simulink model "connections"  (R2020a)
settings: Solver=FixedStepAuto  StartTime=0.0  StopTime=5000  FixedStep=0.1  RelTol=1e-3
values from neighbouring files (symbols this model uses):
  east_drift_limit = 2    [wave_parameters.mat]
  k_down = 1.3    [wave_parameters.mat]
  k_east = 2    [wave_parameters.mat]
  k_north = 2    [wave_parameters.mat]
  k_pitch = 3    [wave_parameters.mat]
  k_roll = 3    [wave_parameters.mat]
  k_yaw = 3    [wave_parameters.mat]
  north_drift_limit = 2    [wave_parameters.mat]
  numberOfBuses = 2    [init.m]
  numberOfGenerators = 4    [init.m]
  peak_frequency = 0.8    [wave_parameters.mat]
  wave_height = 1    [wave_parameters.mat]
  yaw_drift_limit = 0.174532925199    [wave_parameters.mat]
undefined symbols (not defined in the file or in its folder): east, magnitude, north, surge, sway, yaw
libraries: simulink x28, simulink_extras x18
(part 1 of 4)
settings Model: Creator=thomas.evang  LastModifiedBy=thomas.evang
settings RTWCC: Description=Generic Real-Time Target

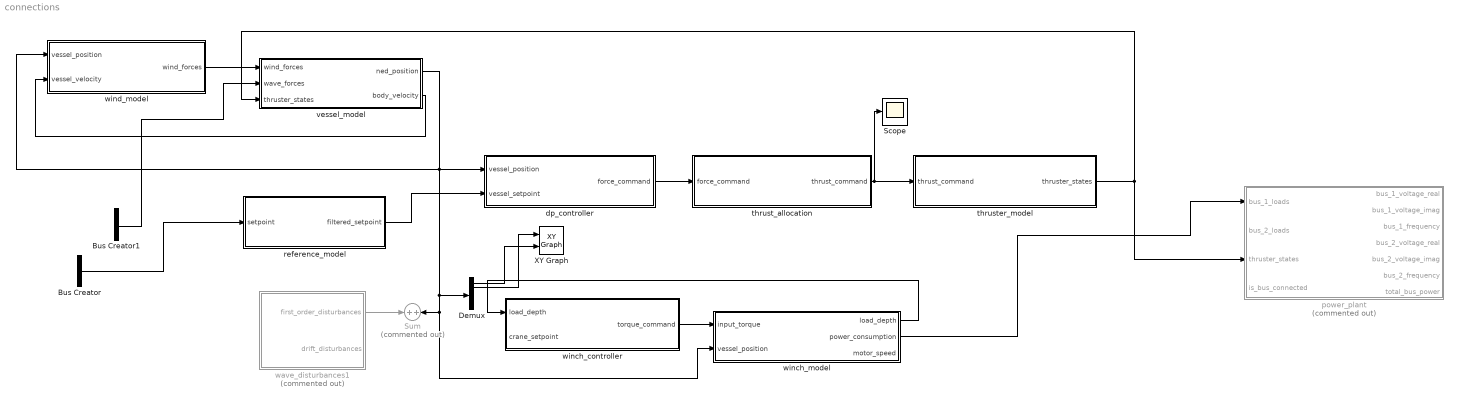
== system connections ==
  Bus Creator : BusCreator  Inputs=3  OutDataTypeStr=Bus: position_3dof
  Bus Creator1 : BusCreator  Inputs=6  OutDataTypeStr=Bus: force_6dof
  Demux : Demux  Outputs=6
  Scope : Scope
  Sum : Sum  Commented=on  Inputs=+|+
  XY Graph : simulink/Sinks/XY Graph  xmin=-20  xmax=20  ymin=-20  ymax=20  st=-1
  dp_controller : Subsystem
  power_plant : Subsystem  Commented=on
  reference_model : Subsystem
  thrust_allocation : Subsystem
  thruster_model : Subsystem
  vessel_model : Subsystem
  wave_disturbances1 : Subsystem  Commented=on  mask{Hs=wave_height, w0=peak_frequency, k_north=k_north, k_east=k_east, k_down=k_down, k_roll=k_roll, k_pitch=k_pitch, k_yaw=k_yaw}
      mask prompts: Hs "Significant Wave Height"; w0 "Peak Frequency"; k_north "North Coefficient"; k_east "East Coefficient"; k_down "Down Coefficient"; k_roll "Roll Coefficient"; k_pitch "Pitch Coefficient"; k_yaw "Yaw Coefficient"
  winch_controller : Subsystem
  winch_model : Subsystem
  wind_model : Subsystem
  wires:
  thrust_allocation/1(thrust_command) -> Scope/1, thruster_model/1(thrust_command)
  dp_controller/1(force_command) -> thrust_allocation/1(force_command)
  reference_model/1(filtered_setpoint) -> dp_controller/2(vessel_setpoint)
  thruster_model/1(thruster_states) -> vessel_model/3(thruster_states), power_plant/3(thruster_states)
  wind_model/1(wind_forces) -> vessel_model/1(wind_forces)
  vessel_model/2(body_velocity) -> wind_model/2(vessel_velocity)
  winch_controller/1(torque_command) -> winch_model/1(input_torque)
  winch_model/1(load_depth) -> winch_controller/1(load_depth)
  winch_model/2(power_consumption) -> power_plant/1(bus_1_loads)
  vessel_model/1(ned_position) -> Demux/1, winch_model/2(vessel_position), Sum/2, dp_controller/1(vessel_position), wind_model/1(vessel_position)
  wave_disturbances1/1(first_order_disturbances) -> Sum/1
  Bus Creator/1 -> reference_model/1(setpoint)
  Bus Creator1/1 -> vessel_model/2(wave_forces)
  ? -> Bus Creator/1
  Demux/2 -> XY Graph/1
  Demux/1 -> XY Graph/2

== system connections/dp_controller ==
  vessel_position : Inport  OutDataTypeStr=Bus: position_6dof
  vessel_setpoint : Inport  Port=2  OutDataTypeStr=Bus: position_3dof
  6DOFRotationMatrix : Subsystem
  Add : Sum  Inputs=-+
  Bus Creator : BusCreator  Inputs=surge,sway,yaw  OutDataTypeStr=Bus: force_3dof
  Bus to Vector : BusToVector
  Bus to Vector1 : BusToVector
  Constant1 : Constant  Value=0
  Demux : Demux  Outputs=3
  Demux1 : Demux  Outputs=3
  Demux2 : Demux  Outputs=3
  Matrix Multiply : Product  Inputs=/*  Multiplication=Matrix(*)
  PID Controller : simulink/Continuous/PID Controller  Controller=PID  Form=Parallel  TimeDomain=Discrete-time  UseExternalTs=off  SampleTime=1e-1  IntegratorMethod=Forward Euler  FilterMethod=Forward Euler  ControllerParametersSource=internal  P=10000  I=0  D=100000  UseFilter=off  N=0  TunerSelectOption=Transfer Function Based (PID Tuner App)  InitialConditionSource=internal  InitialConditionForIntegrator=0  InitialConditionForFilter=0  DifferentiatorICPrevScaledInput=0  ExternalReset=none  TrackingMode=off  Kt=1  LimitOutput=off  UpperSaturationLimit=inf  LowerSaturationLimit=-inf  LinearizeAsGain=on  AntiWindupMode=none  Kb=1  POutMin=[]  POutMax=[]  IOutMin=[]  IOutMax=[]  DOutMin=[]  DOutMax=[]  NOutMin=[]  NOutMax=[]  SumOutMin=[]  SumOutMax=[]  SaturationOutMin=[]  SaturationOutMax=[]  PParamMin=[]  PParamMax=[]  IParamMin=[]  IParamMax=[]  DParamMin=[]  DParamMax=[]  NParamMin=[]  NParamMax=[]  KbParamMin=[]  KbParamMax=[]  KtParamMin=[]  KtParamMax=[]  KbOutMin=[]  KbOutMax=[]  KtOutMin=[]  KtOutMax=[]  IntegratorOutMin=[]  IntegratorOutMax=[]  FilterOutMin=[]  FilterOutMax=[]  SumI1OutMin=[]  SumI1OutMax=[]  SumI2OutMin=[]  SumI2OutMax=[]  SumI3OutMin=[]  SumI3OutMax=[]  SumI4OutMin=[]  SumI4OutMax=[]  SumDOutMin=[]  SumDOutMax=[]  DifferentiatorOutMin=[]  DifferentiatorOutMax=[]  FilterDiffOutCoefMin=[]  FilterDiffOutCoefMax=[]  ReciprocalOutMin=[]  ReciprocalOutMax=[]  SumDenOutMin=[]  SumDenOutMax=[]  SumNumOutMin=[]  SumNumOutMax=[]  DivideOutMin=[]  DivideOutMax=[]  UdiffTsProdOutMin=[]  UdiffTsProdOutMax=[]  NTsProdOutMin=[]  NTsProdOutMax=[]  UintegralTsProdOutMin=[]  UintegralTsProdOutMax=[]  UngainTsProdOutMin=[]  UngainTsProdOutMax=[]  IntegratorContinuousStateAttributes=''  IntegratorStateMustResolveToSignalObject=off  IntegratorRTWStateStorageClass=Auto  FilterContinuousStateAttributes=''  FilterStateMustResolveToSignalObject=off  FilterRTWStateStorageClass=Auto  ParallelPVariant=InternalParameters  IdealPVariant=Disabled  IVariant=InternalParameters  DVariant=InternalParameters  IntegratorVariant=Discrete  SatVariant=Disabled  AWVariant=Passthrough  PCopyVariant=Disabled  TRVariant=Disabled  FdbkBlocksVariant=Forward  IdealPFdbkVariant=Disabled  SatFdbkVariant=Disabled  DerivativeFilterVariant=Differentiator  NVariant=Passthrough  NCopyVariant=Disabled_SignalSpec  FilterICVariant=InternalICsDifferentiator  IntegratorICVariant=InternalICs  ExternalResetVariant=Disabled  TRSumVariant=Passthrough  SumFdbkVariant=Disabled  SumVariant=Sum_PID  TsampFilterVariant=InternalTs  TsampNgainVariant=Passthrough  TsampIntegralVariant=Passthrough
  PID Controller1 : simulink/Continuous/PID Controller  Controller=PID  Form=Parallel  TimeDomain=Discrete-time  UseExternalTs=off  SampleTime=1e-1  IntegratorMethod=Forward Euler  FilterMethod=Forward Euler  ControllerParametersSource=internal  P=10000  I=0  D=100000  UseFilter=off  N=0  TunerSelectOption=Transfer Function Based (PID Tuner App)  InitialConditionSource=internal  InitialConditionForIntegrator=0  InitialConditionForFilter=0  DifferentiatorICPrevScaledInput=0  ExternalReset=none  TrackingMode=off  Kt=1  LimitOutput=off  UpperSaturationLimit=inf  LowerSaturationLimit=-inf  LinearizeAsGain=on  AntiWindupMode=none  Kb=1  POutMin=[]  POutMax=[]  IOutMin=[]  IOutMax=[]  DOutMin=[]  DOutMax=[]  NOutMin=[]  NOutMax=[]  SumOutMin=[]  SumOutMax=[]  SaturationOutMin=[]  SaturationOutMax=[]  PParamMin=[]  PParamMax=[]  IParamMin=[]  IParamMax=[]  DParamMin=[]  DParamMax=[]  NParamMin=[]  NParamMax=[]  KbParamMin=[]  KbParamMax=[]  KtParamMin=[]  KtParamMax=[]  KbOutMin=[]  KbOutMax=[]  KtOutMin=[]  KtOutMax=[]  IntegratorOutMin=[]  IntegratorOutMax=[]  FilterOutMin=[]  FilterOutMax=[]  SumI1OutMin=[]  SumI1OutMax=[]  SumI2OutMin=[]  SumI2OutMax=[]  SumI3OutMin=[]  SumI3OutMax=[]  SumI4OutMin=[]  SumI4OutMax=[]  SumDOutMin=[]  SumDOutMax=[]  DifferentiatorOutMin=[]  DifferentiatorOutMax=[]  FilterDiffOutCoefMin=[]  FilterDiffOutCoefMax=[]  ReciprocalOutMin=[]  ReciprocalOutMax=[]  SumDenOutMin=[]  SumDenOutMax=[]  SumNumOutMin=[]  SumNumOutMax=[]  DivideOutMin=[]  DivideOutMax=[]  UdiffTsProdOutMin=[]  UdiffTsProdOutMax=[]  NTsProdOutMin=[]  NTsProdOutMax=[]  UintegralTsProdOutMin=[]  UintegralTsProdOutMax=[]  UngainTsProdOutMin=[]  UngainTsProdOutMax=[]  IntegratorContinuousStateAttributes=''  IntegratorStateMustResolveToSignalObject=off  IntegratorRTWStateStorageClass=Auto  FilterContinuousStateAttributes=''  FilterStateMustResolveToSignalObject=off  FilterRTWStateStorageClass=Auto  ParallelPVariant=InternalParameters  IdealPVariant=Disabled  IVariant=InternalParameters  DVariant=InternalParameters  IntegratorVariant=Discrete  SatVariant=Disabled  AWVariant=Passthrough  PCopyVariant=Disabled  TRVariant=Disabled  FdbkBlocksVariant=Forward  IdealPFdbkVariant=Disabled  SatFdbkVariant=Disabled  DerivativeFilterVariant=Differentiator  NVariant=Passthrough  NCopyVariant=Disabled_SignalSpec  FilterICVariant=InternalICsDifferentiator  IntegratorICVariant=InternalICs  ExternalResetVariant=Disabled  TRSumVariant=Passthrough  SumFdbkVariant=Disabled  SumVariant=Sum_PID  TsampFilterVariant=InternalTs  TsampNgainVariant=Passthrough  TsampIntegralVariant=Passthrough
  PID Controller2 : simulink/Continuous/PID Controller  Controller=PID  Form=Parallel  TimeDomain=Discrete-time  UseExternalTs=off  SampleTime=1e-1  IntegratorMethod=Forward Euler  FilterMethod=Forward Euler  ControllerParametersSource=internal  P=10000  I=10  D=100000  UseFilter=off  N=100  TunerSelectOption=Transfer Function Based (PID Tuner App)  InitialConditionSource=internal  InitialConditionForIntegrator=0  InitialConditionForFilter=0  DifferentiatorICPrevScaledInput=0  ExternalReset=none  TrackingMode=off  Kt=1  LimitOutput=off  UpperSaturationLimit=inf  LowerSaturationLimit=-inf  LinearizeAsGain=on  AntiWindupMode=none  Kb=1  POutMin=[]  POutMax=[]  IOutMin=[]  IOutMax=[]  DOutMin=[]  DOutMax=[]  NOutMin=[]  NOutMax=[]  SumOutMin=[]  SumOutMax=[]  SaturationOutMin=[]  SaturationOutMax=[]  PParamMin=[]  PParamMax=[]  IParamMin=[]  IParamMax=[]  DParamMin=[]  DParamMax=[]  NParamMin=[]  NParamMax=[]  KbParamMin=[]  KbParamMax=[]  KtParamMin=[]  KtParamMax=[]  KbOutMin=[]  KbOutMax=[]  KtOutMin=[]  KtOutMax=[]  IntegratorOutMin=[]  IntegratorOutMax=[]  FilterOutMin=[]  FilterOutMax=[]  SumI1OutMin=[]  SumI1OutMax=[]  SumI2OutMin=[]  SumI2OutMax=[]  SumI3OutMin=[]  SumI3OutMax=[]  SumI4OutMin=[]  SumI4OutMax=[]  SumDOutMin=[]  SumDOutMax=[]  DifferentiatorOutMin=[]  DifferentiatorOutMax=[]  FilterDiffOutCoefMin=[]  FilterDiffOutCoefMax=[]  ReciprocalOutMin=[]  ReciprocalOutMax=[]  SumDenOutMin=[]  SumDenOutMax=[]  SumNumOutMin=[]  SumNumOutMax=[]  DivideOutMin=[]  DivideOutMax=[]  UdiffTsProdOutMin=[]  UdiffTsProdOutMax=[]  NTsProdOutMin=[]  NTsProdOutMax=[]  UintegralTsProdOutMin=[]  UintegralTsProdOutMax=[]  UngainTsProdOutMin=[]  UngainTsProdOutMax=[]  IntegratorContinuousStateAttributes=''  IntegratorStateMustResolveToSignalObject=off  IntegratorRTWStateStorageClass=Auto  FilterContinuousStateAttributes=''  FilterStateMustResolveToSignalObject=off  FilterRTWStateStorageClass=Auto  ParallelPVariant=InternalParameters  IdealPVariant=Disabled  IVariant=InternalParameters  DVariant=InternalParameters  IntegratorVariant=Discrete  SatVariant=Disabled  AWVariant=Passthrough  PCopyVariant=Disabled  TRVariant=Disabled  FdbkBlocksVariant=Forward  IdealPFdbkVariant=Disabled  SatFdbkVariant=Disabled  DerivativeFilterVariant=Differentiator  NVariant=Passthrough  NCopyVariant=Disabled_SignalSpec  FilterICVariant=InternalICsDifferentiator  IntegratorICVariant=InternalICs  ExternalResetVariant=Disabled  TRSumVariant=Passthrough  SumFdbkVariant=Disabled  SumVariant=Sum_PID  TsampFilterVariant=InternalTs  TsampNgainVariant=Passthrough  TsampIntegralVariant=Passthrough
  Scope : Scope
  Scope1 : Scope
  Scope2 : Scope
  Selector1 : Selector  InputPortWidth=6  IndexOptions=Index vector (dialog)  Indices=[1 2 6]  OutputSizes=1
  Selector2 : Selector  InputPortWidth=6  IndexOptions=Index vector (dialog)  Indices=[1 2 6]  OutputSizes=1
  Selector3 : Selector  InputPortWidth=6  IndexOptions=Index vector (dialog)  Indices=[4 5 6]  OutputSizes=1
  Vector Concatenate : Concatenate  NumInputs=6
  force_command : Outport  OutDataTypeStr=Bus: force_3dof  VectorParamsAs1DForOutWhenUnconnected=off
  wires:
  vessel_position/1 -> Bus to Vector/1
  Selector2/1 -> Demux1/1
  Bus to Vector/1 -> Selector3/1, Selector1/1
  PID Controller1/1 -> Vector Concatenate/2
  Matrix Multiply/1 -> Selector2/1
  Demux1/3 -> Bus Creator/3  "yaw"
  Bus to Vector1/1 -> Add/2
  Selector1/1 -> Add/1
  Demux/1 -> PID Controller/1, Scope1/1  "errorN"
  Demux/2 -> Scope2/1, PID Controller1/1  "errorE"
  Constant1/1 -> Vector Concatenate/5, Vector Concatenate/3, Vector Concatenate/4
  PID Controller2/1 -> Vector Concatenate/6
  6DOFRotationMatrix/1(6DofRotationMatrix) -> Matrix Multiply/1
  Demux1/2 -> Bus Creator/2  "sway"
  Demux/3 -> Scope/1, PID Controller2/1  "errorHeading"
  Bus Creator/1 -> force_command/1
  vessel_setpoint/1 -> Bus to Vector1/1
  Demux1/1 -> Bus Creator/1  "surge"
  Vector Concatenate/1 -> Matrix Multiply/2
  Add/1 -> Demux/1
  PID Controller/1 -> Vector Concatenate/1
  Selector3/1 -> Demux2/1
  Demux2/1 -> 6DOFRotationMatrix/1(roll)
  Demux2/2 -> 6DOFRotationMatrix/2(pitch)
  Demux2/3 -> 6DOFRotationMatrix/3(yaw)

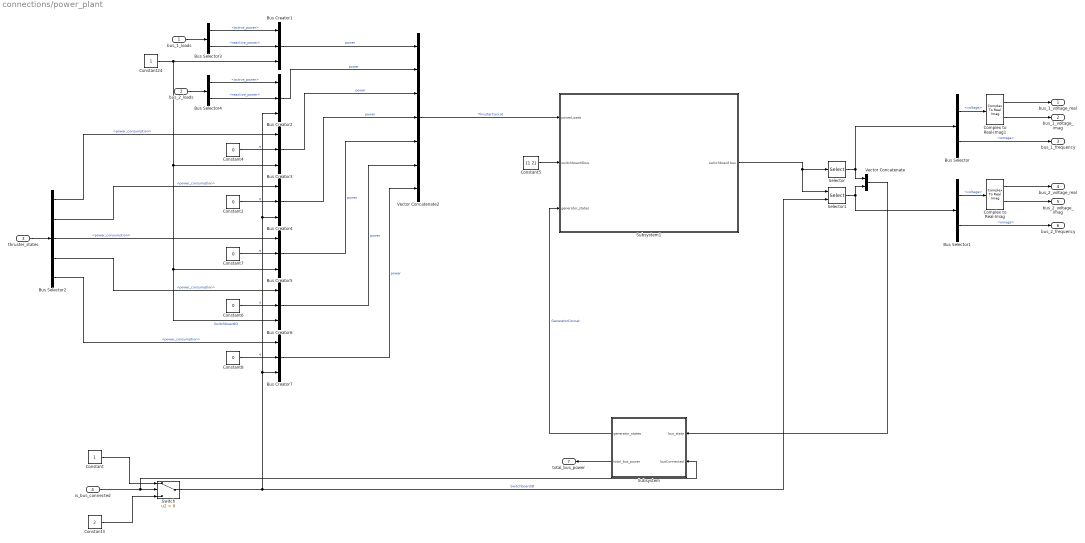
== system connections/power_plant ==
  bus_1_loads : Inport  OutDataTypeStr=Bus: bus_load
  bus_2_loads : Inport  Port=2  OutDataTypeStr=Bus: bus_load
  thruster_states : Inport  Port=3  OutDataTypeStr=Bus: thruster_states
  is_bus_connected : Inport  Port=4  OutDataTypeStr=boolean
  Bus Selector : BusSelector  OutputSignals=voltage,omega
  Bus Selector1 : BusSelector  OutputSignals=voltage,omega
  Bus Selector2 : BusSelector  OutputSignals=tunnel_thruster_1.power_consumption,tunnel_thruster_2.power_consumption,tunnel_thruster_3.power_consumption,main_propeller_port.power_consumption,main_propeller_starboard.power_consumption
  Bus Selector3 : BusSelector  OutputSignals=active_power,reactive_power
  Bus Selector4 : BusSelector  OutputSignals=active_power,reactive_power
  Bus Creator{1..7} (7 alike) : BusCreator  Inputs=3  OutDataTypeStr=Bus: powerLoadsBus  NonVirtualBus=on
      settings: InheritFromInputs=off
  Complex to Real-Imag : ComplexToRealImag
  Complex to Real-Imag1 : ComplexToRealImag
  Constant : Constant
  Constant{2,4,6..8} (5 alike) : Constant  Value=0
  Constant24 : Constant
  Constant3 : Constant  Value=2
  Constant5 : Constant  Value=[1 2]
  Selector : Selector  NumberOfDimensions=2  InputPortWidth=3  IndexOptions=Select all,Index vector (dialog)  Indices=[1 3],1  OutputSizes=1,1
  Selector1 : Selector  NumberOfDimensions=2  InputPortWidth=3  IndexOptions=Select all,Index vector (port)  Indices=[1 3],1  OutputSizes=1,1
  Subsystem : Subsystem
  Subsystem1 : Subsystem
  Switch : Switch  Criteria=u2 > Threshold
  Vector Concatenate : Concatenate  Mode=Multidimensional array  ConcatenateDimension=2
  Vector Concatenate2 : Concatenate  NumInputs=7  Mode=Multidimensional array
  bus_1_voltage_real : Outport  OutDataTypeStr=double  VectorParamsAs1DForOutWhenUnconnected=off
  bus_1_voltage_imag : Outport  Port=2  OutDataTypeStr=double  VectorParamsAs1DForOutWhenUnconnected=off
  bus_1_frequency : Outport  Port=3  OutDataTypeStr=double  VectorParamsAs1DForOutWhenUnconnected=off
  bus_2_voltage_real : Outport  Port=4  OutDataTypeStr=double  VectorParamsAs1DForOutWhenUnconnected=off
  bus_2_voltage_imag : Outport  Port=5  OutDataTypeStr=double  VectorParamsAs1DForOutWhenUnconnected=off
  bus_2_frequency : Outport  Port=6  OutDataTypeStr=double  VectorParamsAs1DForOutWhenUnconnected=off
  total_bus_power : Outport  Port=7  OutDataTypeStr=double  VectorParamsAs1DForOutWhenUnconnected=off
  wires:
  Selector1/1 -> Vector Concatenate/2, Bus Selector1/1
  Bus Selector/1 -> Complex to Real-Imag1/1  "<voltage>"
  Constant24/1 -> Bus Creator6/3, Bus Creator5/3, Bus Creator3/3, Bus Creator1/3  "SwitchboardID"
  Switch/1 -> Bus Creator2/3, Bus Creator4/3, Bus Creator7/3, Selector1/2  "SwitchboardID"
  Constant/1 -> Switch/1
  Subsystem/1(generator_states) -> Subsystem1/3(generator_states)  "GeneratorConcat"
  Bus Creator1/1 -> Vector Concatenate2/1  "power"
  Vector Concatenate2/1 -> Subsystem1/1(powerLoads)  "ThrusterConcat"
  Bus Selector1/2 -> bus_2_frequency/1  "<omega>"
  Subsystem/2(total_bus_power) -> total_bus_power/1
  bus_1_loads/1 -> Bus Selector3/1
  Constant4/1 -> Bus Creator3/2  "q"
  Constant6/1 -> Bus Creator6/2  "q"
  Bus Selector3/1 -> Bus Creator1/1  "<active_power>"
  is_bus_connected/1 -> Subsystem/2(busConnected), Switch/2
  Bus Creator7/1 -> Vector Concatenate2/7  "power"
  bus_2_loads/1 -> Bus Selector4/1
  Subsystem1/1(switchboard bus) -> Selector/1, Selector1/1
  Constant5/1 -> Subsystem1/2(switchboard2bus)
  Bus Selector3/2 -> Bus Creator1/2  "<reactive_power>"
  Bus Selector1/1 -> Complex to Real-Imag/1  "<voltage>"
  Bus Selector2/3 -> Bus Creator5/1  "<power_consumption>"
  Bus Selector2/4 -> Bus Creator6/1  "<power_consumption>"
  Bus Selector4/2 -> Bus Creator2/2  "<reactive_power>"
  Bus Selector2/2 -> Bus Creator4/1  "<power_consumption>"
  Bus Selector2/1 -> Bus Creator3/1  "<power_consumption>"
  Selector/1 -> Vector Concatenate/1, Bus Selector/1
  Vector Concatenate/1 -> Subsystem/1(bus_state)
  Bus Creator6/1 -> Vector Concatenate2/6  "power"
  Bus Creator5/1 -> Vector Concatenate2/5  "power"
  Complex to Real-Imag1/1 -> bus_1_voltage_real/1
  Bus Selector/2 -> bus_1_frequency/1  "<omega>"
  Constant8/1 -> Bus Creator7/2  "q"
  thruster_states/1 -> Bus Selector2/1
  Complex to Real-Imag/2 -> bus_2_voltage_imag/1
  Constant7/1 -> Bus Creator5/2  "q"
  Constant3/1 -> Switch/3
  Bus Creator3/1 -> Vector Concatenate2/3  "power"
  Constant2/1 -> Bus Creator4/2  "q"
  Bus Creator4/1 -> Vector Concatenate2/4  "power"
  Complex to Real-Imag1/2 -> bus_1_voltage_imag/1
  Bus Selector2/5 -> Bus Creator7/1  "<power_consumption>"
  Complex to Real-Imag/1 -> bus_2_voltage_real/1
  Bus Creator2/1 -> Vector Concatenate2/2  "power"
  Bus Selector4/1 -> Bus Creator2/1  "<active_power>"

== system connections/reference_model ==
  setpoint : Inport  OutDataTypeStr=Bus: position_3dof
  Add1 : Sum  Inputs=|+-
  Add2 : Sum  Inputs=|+-
  Bus Creator : BusCreator  Inputs=north,east,yaw  OutDataTypeStr=Bus: position_3dof
  Bus to Vector : BusToVector
  Demux : Demux  Outputs=3
  Gain1 : Gain  Gain=[10 10 20].*[10 10 20]
  Gain2 : Gain  Gain=2*[10 10 20]
  Gain3 : Gain  Gain=[10 10 20].*[10 10 20]
  Integrator : Integrator  InitialCondition=0*1*[1 1 1]  ZeroCross=off
  Integrator1 : Integrator  InitialCondition=0*1*[1 1 1]  ZeroCross=off
  Saturation : Saturate  UpperLimit=1*[1 1 pi/18/6]  LowerLimit=-1*[1 1 pi/18/6]  ZeroCross=off
  Saturation1 : Saturate  UpperLimit=1*[5 5 1]  LowerLimit=-1*[5 5 1]  ZeroCross=off
  filtered_setpoint : Outport  OutDataTypeStr=Bus: position_3dof  VectorParamsAs1DForOutWhenUnconnected=off
  wires:
  Demux/1 -> Bus Creator/1  "north"
  Integrator1/1 -> Gain3/1, Demux/1
  Gain1/1 -> Add2/1
  Saturation1/1 -> Integrator/1
  Add2/1 -> Add1/1
  Saturation/1 -> Integrator1/1
  Integrator/1 -> Gain2/1, Saturation/1
  Gain2/1 -> Add1/2
  Demux/3 -> Bus Creator/3  "yaw"
  Add1/1 -> Saturation1/1
  Gain3/1 -> Add2/2
  Bus to Vector/1 -> Gain1/1
  Demux/2 -> Bus Creator/2  "east"
  setpoint/1 -> Bus to Vector/1
  Bus Creator/1 -> filtered_setpoint/1

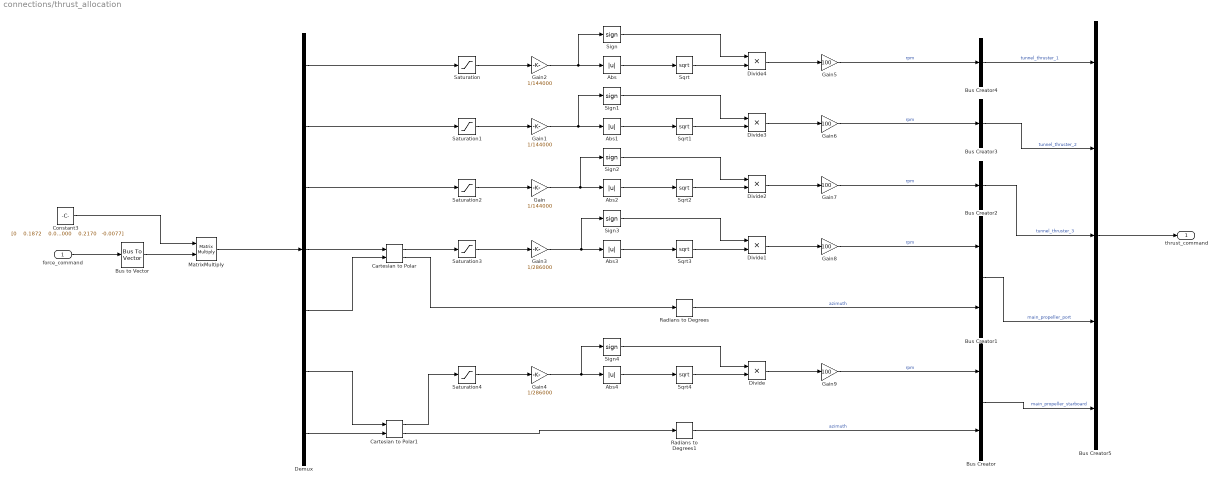
== system connections/thrust_allocation ==
  force_command : Inport  OutDataTypeStr=Bus: force_3dof
  Abs{,1..4} (5 alike) : Abs
  Bus Creator : BusCreator  Inputs=2  OutDataTypeStr=Bus: azimuth_thruster_command
      settings: InheritFromInputs=off
  Bus Creator1 : BusCreator  Inputs=2  OutDataTypeStr=Bus: azimuth_thruster_command
      settings: InheritFromInputs=off
  Bus Creator2 : BusCreator  Inputs=1  OutDataTypeStr=Bus: tunnel_thruster_command
      settings: InheritFromInputs=off
  Bus Creator3 : BusCreator  Inputs=1  OutDataTypeStr=Bus: tunnel_thruster_command
      settings: InheritFromInputs=off
  Bus Creator4 : BusCreator  Inputs=1  OutDataTypeStr=Bus: tunnel_thruster_command
      settings: InheritFromInputs=off
  Bus Creator5 : BusCreator  Inputs=5  OutDataTypeStr=Bus: thrust_command
      settings: InheritFromInputs=off
  Bus to Vector : BusToVector
  Cartesian to Polar : simulink_extras/Transformations/Cartesian to Polar
  Cartesian to Polar1 : simulink_extras/Transformations/Cartesian to Polar
  Constant3 : Constant  Value=|
      | [0    0.1872    0.0058;
      |     0.0000    0.1886    0.0051;
      |     0.0000    0.1901    0.0045;
      |     0.5000   -0.0018    0.0008;
      |     0.0000    0.2170   -0.0077;
      |     0.5000    0.0018   -0.0008;
      |     0.0000    0.2170   -0.0077]
  Demux : Demux  Outputs=7
  Divide{,1..4} (5 alike) : Product
  Gain : Gain  Gain=1/144000
  Gain1 : Gain  Gain=1/144000
  Gain2 : Gain  Gain=1/144000
  Gain3 : Gain  Gain=1/286000
  Gain4 : Gain  Gain=1/286000
  Gain{5..9} (5 alike) : Gain  Gain=100
  MatrixMultiply : Product  Multiplication=Matrix(*)
  Radians to Degrees : simulink_extras/Transformations/Radians to Degrees
  Radians to Degrees1 : simulink_extras/Transformations/Radians to Degrees
  Saturation : Saturate  UpperLimit=144000  LowerLimit=-144000
  Saturation1 : Saturate  UpperLimit=144000  LowerLimit=-144000
  Saturation2 : Saturate  UpperLimit=144000  LowerLimit=-144000
  Saturation3 : Saturate  UpperLimit=286000  LowerLimit=0
  Saturation4 : Saturate  UpperLimit=286000  LowerLimit=0
  Sign{,1..4} (5 alike) : Signum
  Sqrt{,1..4} (5 alike) : Sqrt  SaturateOnIntegerOverflow=on
  thrust_command : Outport  OutDataTypeStr=Bus: thrust_command  VectorParamsAs1DForOutWhenUnconnected=off
  wires:
  Saturation2/1 -> Gain/1
  Constant3/1 -> MatrixMultiply/1
  Abs1/1 -> Sqrt1/1
  MatrixMultiply/1 -> Demux/1
  Gain1/1 -> Sign1/1, Abs1/1
  Saturation3/1 -> Gain3/1
  Gain2/1 -> Sign/1, Abs/1
  Sign2/1 -> Divide2/1
  Sign/1 -> Divide4/1
  Bus Creator5/1 -> thrust_command/1
  Demux/2 -> Saturation1/1
  Bus to Vector/1 -> MatrixMultiply/2
  Saturation1/1 -> Gain1/1
  Bus Creator3/1 -> Bus Creator5/2  "tunnel_thruster_2"
  Bus Creator2/1 -> Bus Creator5/3  "tunnel_thruster_3"
  Bus Creator4/1 -> Bus Creator5/1  "tunnel_thruster_1"
  Abs4/1 -> Sqrt4/1
  Sqrt/1 -> Divide4/2
  Demux/1 -> Saturation/1
  Bus Creator/1 -> Bus Creator5/5  "main_propeller_starboard"
  Gain/1 -> Sign2/1, Abs2/1
  Demux/4 -> Cartesian to Polar/1
  Sqrt1/1 -> Divide3/2
  Sign4/1 -> Divide/1
  Gain8/1 -> Bus Creator1/1  "rpm"
  Gain5/1 -> Bus Creator4/1  "rpm"
  Divide1/1 -> Gain8/1
  Gain6/1 -> Bus Creator3/1  "rpm"
  force_command/1 -> Bus to Vector/1
  Cartesian to Polar/1 -> Saturation3/1
  Sqrt2/1 -> Divide2/2
  Abs3/1 -> Sqrt3/1
  Cartesian to Polar1/1 -> Saturation4/1
  Divide2/1 -> Gain7/1
  Gain3/1 -> Sign3/1, Abs3/1
  Gain9/1 -> Bus Creator/1  "rpm"
  Sign1/1 -> Divide3/1
  Radians to Degrees1/1 -> Bus Creator/2  "azimuth"
  Demux/5 -> Cartesian to Polar/2
  Demux/6 -> Cartesian to Polar1/1
  Bus Creator1/1 -> Bus Creator5/4  "main_propeller_port"
  Demux/3 -> Saturation2/1
  Divide3/1 -> Gain6/1
  Sqrt3/1 -> Divide1/2
  Divide/1 -> Gain9/1
  Divide4/1 -> Gain5/1
  Saturation/1 -> Gain2/1
  Radians to Degrees/1 -> Bus Creator1/2  "azimuth"
  Demux/7 -> Cartesian to Polar1/2
  Abs2/1 -> Sqrt2/1
  Gain4/1 -> Sign4/1, Abs4/1
  Sqrt4/1 -> Divide/2
  Abs/1 -> Sqrt/1
  Saturation4/1 -> Gain4/1
  Gain7/1 -> Bus Creator2/1  "rpm"
  Sign3/1 -> Divide1/1
  Cartesian to Polar1/2 -> Radians to Degrees1/1
  Cartesian to Polar/2 -> Radians to Degrees/1

== system connections/thruster_model ==
  note: MPPS
  note: TT1
  note: TT1
  note: TT3
  note: TT2
  note: MPSB
  thrust_command : Inport  OutDataTypeStr=Bus: thrust_command
  Bus Creator : BusCreator  Inputs=3
  Bus Creator1 : BusCreator  Inputs=3
  Bus Creator2 : BusCreator  Inputs=2
  Bus Creator3 : BusCreator  Inputs=2
  Bus Creator4 : BusCreator  Inputs=2
  Bus Creator5 : BusCreator  Inputs=5  OutDataTypeStr=Bus: thruster_states
  Bus to Vector : BusToVector
  Constant : Constant  Value=90
  Demux : Demux  Outputs=7
  Terminator{,1..7} (8 alike) : Terminator
  main_propeller_port : Subsystem
  main_propeller_starboard : Subsystem
  tunnel_thruster_1 : Subsystem
  tunnel_thruster_2 : Subsystem
  tunnel_thruster_3 : Subsystem
  thruster_states : Outport  OutDataTypeStr=Bus: thruster_states  VectorParamsAs1DForOutWhenUnconnected=off
  wires:
  tunnel_thruster_1/2(thrust) -> Bus Creator4/2  "thrust"
  main_propeller_starboard/1(p) -> Bus Creator1/1  "power_consumption"
  Bus Creator3/1 -> Bus Creator5/2  "tunnel_thruster_2"
  Demux/7 -> main_propeller_starboard/2(desiredAzimuth)
  Bus Creator2/1 -> Bus Creator5/3  "tunnel_thruster_3"
  main_propeller_starboard/3(azimuth) -> Bus Creator1/3  "azimuth"
  tunnel_thruster_1/3(azimuth) -> Terminator6/1
  main_propeller_port/2(thrust) -> Bus Creator/2  "thrust"
  tunnel_thruster_2/2(thrust) -> Bus Creator3/2  "thrust"
  tunnel_thruster_1/1(p) -> Bus Creator4/1  "power_consumption"
  Demux/3 -> tunnel_thruster_3/1(desiredSetPoint)
  Demux/6 -> main_propeller_starboard/1(desiredSetPoint)
  Bus Creator4/1 -> Bus Creator5/1  "tunnel_thruster_1"
  tunnel_thruster_1/4(sensorFeedback) -> Terminator7/1
  tunnel_thruster_3/1(p) -> Bus Creator2/1  "power_consumption"
  tunnel_thruster_2/1(p) -> Bus Creator3/1  "power_consumption"
  main_propeller_port/1(p) -> Bus Creator/1  "power_consumption"
  tunnel_thruster_3/2(thrust) -> Bus Creator2/2  "thrust"
  Bus Creator1/1 -> Bus Creator5/5  "main_propeller_starboard"
  tunnel_thruster_3/3(azimuth) -> Terminator2/1
  Bus Creator/1 -> Bus Creator5/4  "main_propeller_port"
  Demux/2 -> tunnel_thruster_2/1(desiredSetPoint)
  main_propeller_port/3(azimuth) -> Bus Creator/3  "azimuth"
  main_propeller_port/4(sensorFeedback) -> Terminator1/1
  Bus Creator5/1 -> thruster_states/1
  main_propeller_starboard/4(sensorFeedback) -> Terminator/1
  tunnel_thruster_2/4(sensorFeedback) -> Terminator5/1
  Demux/5 -> main_propeller_port/2(desiredAzimuth)
  thrust_command/1 -> Bus to Vector/1
  tunnel_thruster_3/4(sensorFeedback) -> Terminator3/1
  main_propeller_starboard/2(thrust) -> Bus Creator1/2  "thrust"
  Demux/4 -> main_propeller_port/1(desiredSetPoint)
  Constant/1 -> tunnel_thruster_3/2(desiredAzimuth), tunnel_thruster_2/2(desiredAzimuth), tunnel_thruster_1/2(desiredAzimuth)
  Bus to Vector/1 -> Demux/1
  Demux/1 -> tunnel_thruster_1/1(desiredSetPoint)
  tunnel_thruster_2/3(azimuth) -> Terminator4/1

== system connections/vessel_model ==
  wind_forces : Inport  OutDataTypeStr=Bus: force_6dof
  wave_forces : Inport  Port=2  OutDataTypeStr=Bus: force_6dof
  thruster_states : Inport  Port=3  OutDataTypeStr=Bus: thruster_states
  Add : Sum  Inputs=+++|
  Bus Creator : BusCreator  Inputs=6  OutDataTypeStr=Bus: position_6dof
  Bus Creator2 : BusCreator  Inputs=6  OutDataTypeStr=Bus: velocity_6dof
  Bus Selector : BusSelector  OutputSignals=tunnel_thruster_1,tunnel_thruster_2,tunnel_thruster_3,main_propeller_port,main_propeller_starboard
  Bus to Vector : BusToVector
  Bus to Vector1 : BusToVector
  Demux : Demux  Outputs=6
  Demux1 : Demux  Outputs=6
  VesselDynamics : Subsystem
  thrust_to_forces : Subsystem
  ned_position : Outport  OutDataTypeStr=Bus: position_6dof  VectorParamsAs1DForOutWhenUnconnected=off
  body_velocity : Outport  Port=2  OutDataTypeStr=Bus: velocity_6dof  VectorParamsAs1DForOutWhenUnconnected=off
  wires:
  thrust_to_forces/1(ForcesAndMomentsvector) -> Add/3
  thruster_states/1 -> Bus Selector/1
  Bus Selector/5 -> thrust_to_forces/5(main_propeller_starboard)  "<main_propeller_starboard>"
  Demux1/2 -> Bus Creator2/2
  Add/1 -> VesselDynamics/1(ExternalForceAndMoments)
  Demux/1 -> Bus Creator/1
  Demux/5 -> Bus Creator/5
  Bus Selector/3 -> thrust_to_forces/3(tunnel_thruster_3)  "<tunnel_thruster_3>"
  Demux1/5 -> Bus Creator2/5
  Bus Selector/1 -> thrust_to_forces/1(tunnel_thruster_1)  "<tunnel_thruster_1>"
  Bus Creator/1 -> ned_position/1
  Demux/4 -> Bus Creator/4
  Bus Creator2/1 -> body_velocity/1
  Bus Selector/2 -> thrust_to_forces/2(tunnel_thruster_2)  "<tunnel_thruster_2>"
  VesselDynamics/2(nu) -> Demux1/1  "body_velocity"
  Demux/3 -> Bus Creator/3
  Demux/2 -> Bus Creator/2
  Demux1/1 -> Bus Creator2/1
  Demux1/6 -> Bus Creator2/6
  Bus to Vector/1 -> Add/1
  Bus Selector/4 -> thrust_to_forces/4(main_propeller_port)  "<main_propeller_port>"
  Demux1/3 -> Bus Creator2/3
  wind_forces/1 -> Bus to Vector/1
  Bus to Vector1/1 -> Add/2
  VesselDynamics/1(eta) -> Demux/1  "ned_position"
  Demux1/4 -> Bus Creator2/4
  Demux/6 -> Bus Creator/6
  wave_forces/1 -> Bus to Vector1/1

== system connections/wave_disturbances1 ==
  Band-Limited White Noise : simulink/Sources/Band-Limited White Noise  Cov=[0.005]  Ts=0.1  seed=[23341]
  Band-Limited White Noise1 : simulink/Sources/Band-Limited White Noise  Cov=[0.005]  Ts=0.1  seed=[23341]
  Band-Limited White Noise2 : simulink/Sources/Band-Limited White Noise  Cov=[0.005]  Ts=0.1  seed=[23341]
  Bus Creator : BusCreator  Inputs=6  OutDataTypeStr=Bus: position_6dof
      settings: InheritFromInputs=off
  Constant : Constant  Value=wave_height
  Constant1 : Constant  Value=0
  Mux : Mux  Inputs=6
  Scope : Scope
  east_drift : Integrator  LimitOutput=on  UpperSaturationLimit=east_drift_limit  LowerSaturationLimit=-east_drift_limit
  k_down : Gain  Gain=k_down
  k_east : Gain  Gain=k_east
  k_north : Gain  Gain=k_north
  k_pitch : Gain  Gain=k_pitch
  k_roll : Gain  Gain=k_roll
  k_yaw : Gain  Gain=k_yaw
  north_drift : Integrator  LimitOutput=on  UpperSaturationLimit=north_drift_limit  LowerSaturationLimit=-north_drift_limit
  wave_response5 : Subsystem  mask{w0=peak_frequency}
      mask prompts: w0 "Peak Frequency"
  wave_response_down : Subsystem  mask{w0=peak_frequency}
      mask prompts: w0 "Peak Frequency"
  wave_response_east : Subsystem  mask{w0=peak_frequency}
      mask prompts: w0 "Peak Frequency"
  wave_response_north : Subsystem  mask{w0=peak_frequency}
      mask prompts: w0 "Peak Frequency"
  wave_response_pitch : Subsystem  mask{w0=peak_frequency}
      mask prompts: w0 "Peak Frequency"
  wave_response_roll : Subsystem  mask{w0=peak_frequency}
      mask prompts: w0 "Peak Frequency"
  yaw_drift : Integrator  LimitOutput=on  UpperSaturationLimit=yaw_drift_limit  LowerSaturationLimit=-yaw_drift_limit
  first_order_disturbances : Outport
  drift_disturbances : Outport  Port=2
  wires:
  k_pitch/1 -> Mux/5
  k_yaw/1 -> Scope/1, Mux/6
  Mux/1 -> first_order_disturbances/1
  k_north/1 -> Mux/1
  k_down/1 -> Mux/3
  k_east/1 -> Mux/2
  k_roll/1 -> Mux/4
  Constant/1 -> wave_response_north/1(Hs), wave_response_east/1(Hs), wave_response_down/1(Hs), wave_response_roll/1(Hs), wave_response_pitch/1(Hs), wave_response5/1(Hs)
  wave_response_north/1(Out1) -> k_north/1
  wave_response_east/1(Out1) -> k_east/1
  wave_response_down/1(Out1) -> k_down/1
  wave_response_roll/1(Out1) -> k_roll/1
  wave_response_pitch/1(Out1) -> k_pitch/1
  wave_response5/1(Out1) -> k_yaw/1
  north_drift/1 -> Bus Creator/1
  east_drift/1 -> Bus Creator/2
  Bus Creator/1 -> drift_disturbances/1
  yaw_drift/1 -> Bus Creator/6
  Constant1/1 -> Bus Creator/5, Bus Creator/4, Bus Creator/3
  Band-Limited White Noise1/1 -> east_drift/1
  Band-Limited White Noise2/1 -> yaw_drift/1
  Band-Limited White Noise/1 -> north_drift/1

== system connections/winch_controller ==
  load_depth : Inport
  crane_setpoint : Inport  Port=2
  Add1 : Sum  Inputs=|+-
  Memory : Memory  InitialCondition=500
  PID Controller1 : simulink/Continuous/PID Controller  Controller=PID  Form=Parallel  TimeDomain=Discrete-time  UseExternalTs=off  SampleTime=1e-1  IntegratorMethod=Forward Euler  FilterMethod=Forward Euler  ControllerParametersSource=internal  P=200  I=1  D=1000  UseFilter=off  N=100  TunerSelectOption=Transfer Function Based (PID Tuner App)  ZeroCross=off  InitialConditionSource=internal  InitialConditionForIntegrator=0  InitialConditionForFilter=0  DifferentiatorICPrevScaledInput=0  ExternalReset=none  TrackingMode=off  Kt=1  LimitOutput=off  UpperSaturationLimit=inf  LowerSaturationLimit=-inf  LinearizeAsGain=on  AntiWindupMode=none  Kb=1  POutMin=[]  POutMax=[]  IOutMin=[]  IOutMax=[]  DOutMin=[]  DOutMax=[]  NOutMin=[]  NOutMax=[]  SumOutMin=[]  SumOutMax=[]  SaturationOutMin=[]  SaturationOutMax=[]  PParamMin=[]  PParamMax=[]  IParamMin=[]  IParamMax=[]  DParamMin=[]  DParamMax=[]  NParamMin=[]  NParamMax=[]  KbParamMin=[]  KbParamMax=[]  KtParamMin=[]  KtParamMax=[]  KbOutMin=[]  KbOutMax=[]  KtOutMin=[]  KtOutMax=[]  IntegratorOutMin=[]  IntegratorOutMax=[]  FilterOutMin=[]  FilterOutMax=[]  SumI1OutMin=[]  SumI1OutMax=[]  SumI2OutMin=[]  SumI2OutMax=[]  SumI3OutMin=[]  SumI3OutMax=[]  SumI4OutMin=[]  SumI4OutMax=[]  SumDOutMin=[]  SumDOutMax=[]  DifferentiatorOutMin=[]  DifferentiatorOutMax=[]  FilterDiffOutCoefMin=[]  FilterDiffOutCoefMax=[]  ReciprocalOutMin=[]  ReciprocalOutMax=[]  SumDenOutMin=[]  SumDenOutMax=[]  SumNumOutMin=[]  SumNumOutMax=[]  DivideOutMin=[]  DivideOutMax=[]  UdiffTsProdOutMin=[]  UdiffTsProdOutMax=[]  NTsProdOutMin=[]  NTsProdOutMax=[]  UintegralTsProdOutMin=[]  UintegralTsProdOutMax=[]  UngainTsProdOutMin=[]  UngainTsProdOutMax=[]  IntegratorContinuousStateAttributes=''  IntegratorStateMustResolveToSignalObject=off  IntegratorRTWStateStorageClass=Auto  FilterContinuousStateAttributes=''  FilterStateMustResolveToSignalObject=off  FilterRTWStateStorageClass=Auto  ParallelPVariant=InternalParameters  IdealPVariant=Disabled  IVariant=InternalParameters  DVariant=InternalParameters  IntegratorVariant=Discrete  SatVariant=Disabled  AWVariant=Passthrough  PCopyVariant=Disabled  TRVariant=Disabled  FdbkBlocksVariant=Forward  IdealPFdbkVariant=Disabled  SatFdbkVariant=Disabled  DerivativeFilterVariant=Differentiator  NVariant=Passthrough  NCopyVariant=Disabled_SignalSpec  FilterICVariant=InternalICsDifferentiator  IntegratorICVariant=InternalICs  ExternalResetVariant=Disabled  TRSumVariant=Passthrough  SumFdbkVariant=Disabled  SumVariant=Sum_PID  TsampFilterVariant=InternalTs  TsampNgainVariant=Passthrough  TsampIntegralVariant=Passthrough
  referenceModel : Subsystem
  torque_command : Outport  VectorParamsAs1DForOutWhenUnconnected=off
  wires:
  referenceModel/1(Out1) -> Add1/1  "SetPointSmooth"
  Add1/1 -> PID Controller1/1
  crane_setpoint/1 -> referenceModel/1(In1)
  PID Controller1/1 -> torque_command/1  "forcePID"
  load_depth/1 -> Memory/1
  Memory/1 -> Add1/2

== system connections/winch_model ==
  input_torque : Inport  OutDataTypeStr=double
  vessel_position : Inport  Port=2  OutDataTypeStr=Bus: position_6dof
  Add2 : Sum  Inputs=++|
  Add3 : Sum  Inputs=|++
  Bus to Vector : BusToVector
  ConstantForces : Constant  Value=2.513027
  Divide : Product  Inputs=**
  Gain1 : Gain  Gain=0.0013712275
  Gain2 : Gain  Gain=77.7
  Integrator : Integrator
  Integrator1 : Integrator  InitialCondition=500
  Selector2 : Selector  InputPortWidth=6  IndexOptions=Index vector (dialog)  Indices=3  OutputSizes=1
  Unary Minus1 : UnaryMinus
  load_depth : Outport  VectorParamsAs1DForOutWhenUnconnected=off
  power_consumption : Outport  Port=2  VectorParamsAs1DForOutWhenUnconnected=off
  motor_speed : Outport  Port=3  VectorParamsAs1DForOutWhenUnconnected=off
  wires:
  Integrator1/1 -> Add3/1
  Gain2/1 -> motor_speed/1, Divide/2  "modelMotorSpeed"
  Unary Minus1/1 -> Add3/2
  Add3/1 -> load_depth/1  "modelLoadDepth"
  input_torque/1 -> Divide/1, Gain1/1
  Bus to Vector/1 -> Selector2/1
  ConstantForces/1 -> Add2/2
  Gain1/1 -> Add2/1
  vessel_position/1 -> Bus to Vector/1
  Add2/1 -> Integrator/1
  Integrator/1 -> Gain2/1, Integrator1/1
  Divide/1 -> power_consumption/1  "Power"
  Selector2/1 -> Unary Minus1/1

== system connections/wind_model ==
  vessel_position : Inport  OutDataTypeStr=Bus: position_6dof
  vessel_velocity : Inport  Port=2  OutDataTypeStr=Bus: velocity_6dof
  Bus Creator : BusCreator  Inputs=6  OutDataTypeStr=Bus: force_6dof
      settings: InheritFromInputs=off
  Bus to Vector : BusToVector
  Bus to Vector1 : BusToVector
  Demux : Demux  Outputs=6
  Selector1 : Selector  InputPortWidth=6  IndexOptions=Index vector (dialog)  Indices=2  OutputSizes=1
  Selector2 : Selector  InputPortWidth=6  IndexOptions=Index vector (dialog)  Indices=1  OutputSizes=1
  Selector3 : Selector  InputPortWidth=6  IndexOptions=Index vector (dialog)  Indices=6  OutputSizes=1
  Subsystem : Subsystem
  Subsystem1 : Subsystem  mask{uMean=10, thetaMeanDegrees=0}
      mask prompts: uMean "Mean Wind Speed"; thetaMeanDegrees "Mean Wind Direction"
  wind_forces : Outport  OutDataTypeStr=Bus: force_6dof  VectorParamsAs1DForOutWhenUnconnected=off
  wires:
  Demux/3 -> Bus Creator/3
  Subsystem1/2(wind_direction) -> Subsystem/2(wind direction (NED degrees))
  Subsystem1/1(wind_speed) -> Subsystem/1(wind speed)
  Demux/1 -> Bus Creator/1
  Bus to Vector1/1 -> Selector3/1
  vessel_position/1 -> Bus to Vector1/1
  Selector3/1 -> Subsystem/5(vessel direction (NED degrees))
  Subsystem/1(forcesAndMoments) -> Demux/1  "windForces"
  Demux/6 -> Bus Creator/6
  vessel_velocity/1 -> Bus to Vector/1
  Selector2/1 -> Subsystem/3(vessel surge speed)
  Bus to Vector/1 -> Selector1/1, Selector2/1
  Demux/2 -> Bus Creator/2
  Selector1/1 -> Subsystem/4(vessel sway speed)
  Demux/4 -> Bus Creator/4
  Demux/5 -> Bus Creator/5
  Bus Creator/1 -> wind_forces/1

== system connections/dp_controller/6DOFRotationMatrix ==
  roll : Inport
  pitch : Inport  Port=2
  yaw : Inport  Port=3
  J1 : Subsystem
  J2 : Subsystem
  Matrix Concatenate : Concatenate  Mode=Multidimensional array
  Matrix Concatenate1 : Concatenate  Mode=Multidimensional array
  Matrix Concatenate2 : Concatenate  Mode=Multidimensional array  ConcatenateDimension=2
  Zeros : Constant  Value=zeros(3,3)
  6DofRotationMatrix : Outport  VectorParamsAs1DForOutWhenUnconnected=off
  wires:
  J1/1(linear rotation matrix) -> Matrix Concatenate/1
  yaw/1 -> J1/1(yaw)
  J2/1(angular rotation matrix) -> Matrix Concatenate1/2
  Matrix Concatenate2/1 -> 6DofRotationMatrix/1
  Matrix Concatenate/1 -> Matrix Concatenate2/1
  Matrix Concatenate1/1 -> Matrix Concatenate2/2
  Zeros/1 -> Matrix Concatenate1/1, Matrix Concatenate/2
  roll/1 -> J2/2(roll angle), J1/3(roll)
  pitch/1 -> J1/2(pitch), J2/1(pitch angle)

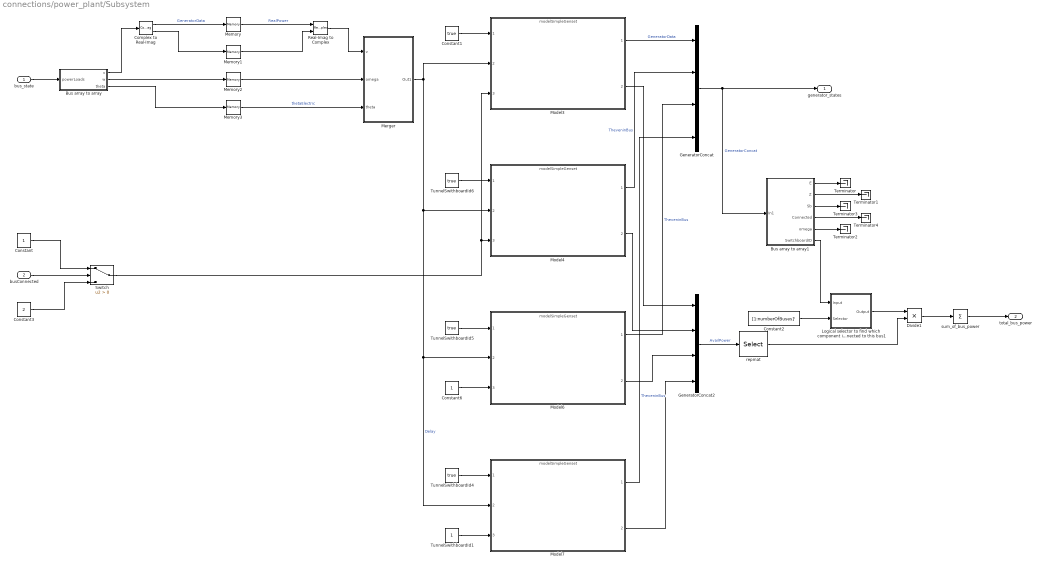
== system connections/power_plant/Subsystem ==
  bus_state : Inport
  busConnected : Inport  Port=2
  Bus array to array : Subsystem  TreatAsAtomicUnit=on
  Bus array to array1 : Subsystem  TreatAsAtomicUnit=on
  Complex to Real-Imag : ComplexToRealImag
  Constant : Constant
  Constant1 : Constant  Value=true
  Constant2 : Constant  Value=[1:numberOfBuses]'  VectorParams1D=off
  Constant3 : Constant  Value=2
  Constant6 : Constant
  Divide1 : Product
  GeneratorConcat : Concatenate  NumInputs=4  Mode=Multidimensional array
  GeneratorConcat2 : Concatenate  NumInputs=4  Mode=Multidimensional array
  Logical selector to find which component is connected to this bus1 : Subsystem
  Memory : Memory  InitialCondition=0.7
  Memory1 : Memory  InitialCondition=0.7
  Memory2 : Memory  InitialCondition=1
  Memory3 : Memory  InitialCondition=pi/4
  Merger : Subsystem  TreatAsAtomicUnit=on
  Model3 : ModelReference  ModelNameDialog=modelSimpleGenset.slx  ParameterArgumentNames=ratedPower  ParameterArgumentValues=[3000000]  UsingDefaultArgumentValue=0  SimulationMode=Normal  ModelReferenceVersion=1.210
  Model4 : ModelReference  ModelNameDialog=modelSimpleGenset.slx  ParameterArgumentNames=ratedPower  ParameterArgumentValues=3000000  UsingDefaultArgumentValue=0  SimulationMode=Normal  ModelReferenceVersion=1.210
  Model6 : ModelReference  ModelNameDialog=modelSimpleGenset.slx  ParameterArgumentNames=ratedPower  ParameterArgumentValues=3000000  UsingDefaultArgumentValue=0  SimulationMode=Normal  ModelReferenceVersion=1.210
  Model7 : ModelReference  ModelNameDialog=modelSimpleGenset.slx  ParameterArgumentNames=ratedPower  ParameterArgumentValues=3000000  UsingDefaultArgumentValue=0  SimulationMode=Normal  ModelReferenceVersion=1.210
  Real-Imag to Complex : RealImagToComplex
  Switch : Switch  Criteria=u2 > Threshold
  Terminator{,1..4} (5 alike) : Terminator
  TunnelSwithboardId1 : Constant
  TunnelSwithboardId4 : Constant  Value=true
  TunnelSwithboardId5 : Constant  Value=true
  TunnelSwithboardId6 : Constant  Value=true
  repmat : Selector  NumberOfDimensions=2  IndexOptions=Index vector (dialog),Index vector (dialog)  Indices=-1,ones(1,numberOfBuses)  OutputSizes=1,1
  sum_of_bus_power : Sum  Inputs=+  CollapseMode=Specified dimension
  generator_states : Outport  VectorParamsAs1DForOutWhenUnconnected=off
  total_bus_power : Outport  Port=2  VectorParamsAs1DForOutWhenUnconnected=off
  wires:
  Bus array to array/2(w) -> Memory2/1
  TunnelSwithboardId1/1 -> Model7/3
  Bus array to array/1(v) -> Complex to Real-Imag/1
  Real-Imag to Complex/1 -> Merger/1(v)
  Model3/1 -> GeneratorConcat/1  "GeneratorData"
  Model4/1 -> GeneratorConcat/2  "TheveninBus"
  Memory3/1 -> Merger/3(theta)  "thetaElectric"
  Merger/1(Out1) -> Model3/2, Model4/2, Model7/2, Model6/2  "Delay"
  Memory/1 -> Real-Imag to Complex/1  "RealPower"
  Memory1/1 -> Real-Imag to Complex/2
  Model6/1 -> GeneratorConcat/3  "TheveninBus"
  Memory2/1 -> Merger/2(omega)
  Model7/1 -> GeneratorConcat/4  "TheveninBus"
  Complex to Real-Imag/1 -> Memory/1  "GeneratorData"
  Complex to Real-Imag/2 -> Memory1/1
  Switch/1 -> Model4/3, Model3/3
  Bus array to array/3(theta) -> Memory3/1
  Constant6/1 -> Model6/3
  bus_state/1 -> Bus array to array/1(powerLoads)
  GeneratorConcat/1 -> Bus array to array1/1(In1), generator_states/1  "GeneratorConcat"
  Constant1/1 -> Model3/1
  TunnelSwithboardId6/1 -> Model4/1
  TunnelSwithboardId5/1 -> Model6/1
  TunnelSwithboardId4/1 -> Model7/1
  Bus array to array1/1(E) -> Terminator/1
  Bus array to array1/2(Z) -> Terminator1/1
  Bus array to array1/5(omega) -> Terminator2/1
  Bus array to array1/6(SwitchboardID) -> Logical selector to find which component is connected to this bus1/1(Input)
  Constant2/1 -> Logical selector to find which component is connected to this bus1/2(Selector)
  Model3/2 -> GeneratorConcat2/1
  Model4/2 -> GeneratorConcat2/2
  Model6/2 -> GeneratorConcat2/3
  Model7/2 -> GeneratorConcat2/4
  GeneratorConcat2/1 -> repmat/1  "AvailPower"
  Logical selector to find which component is connected to this bus1/1(Output) -> Divide1/1
  repmat/1 -> Divide1/2
  Divide1/1 -> sum_of_bus_power/1
  sum_of_bus_power/1 -> total_bus_power/1
  Bus array to array1/4(Connected) -> Terminator4/1
  Bus array to array1/3(Sb) -> Terminator3/1
  busConnected/1 -> Switch/2
  Constant/1 -> Switch/1
  Constant3/1 -> Switch/3

== system connections/power_plant/Subsystem1 ==
  powerLoads : Inport  OutDataTypeStr=Bus: powerLoadsBus  PortDimensions=[7, 1]  BusOutputAsStruct=on
  switchboard2bus : Inport  Port=2
  generator_states : Inport  Port=3  OutDataTypeStr=Bus: TheveninBus  PortDimensions=[4, 1]  BusOutputAsStruct=on
  Constant2 : Constant  Value=-1
  Integrator : Integrator
  MATLAB Function1 : MATLAB Function  Commented=on  TreatAsAtomicUnit=on
  Saturation : Saturate  UpperLimit=0  LowerLimit=-1
  Subsystem1 : Subsystem
  Subsystem2 : Subsystem
  Sum : Sum  Inputs=++|
  thrustersToBuses : Subsystem
  switchboard bus : Outport  OutDataTypeStr=Bus: swb  VectorParamsAs1DForOutWhenUnconnected=off  BusOutputAsStruct=on
  wires:
  Constant2/1 -> Sum/1
  Integrator/1 -> MATLAB Function1/1(u)
  Sum/1 -> Saturation/1
  Saturation/1 -> Integrator/1
  thrustersToBuses/1(loads) -> Subsystem2/1(loads)
  switchboard2bus/1 -> Subsystem1/1(switchboard2bus), Subsystem2/2(switchboard2bus), thrustersToBuses/2(s2b)  "s2b"
  generator_states/1 -> Subsystem1/2(Generatorset)  "Generatorset"
  Subsystem1/1(switchboard bus) -> Subsystem2/3(switchboardBus)
  Subsystem2/1(switchboard bus) -> switchboard bus/1
  Subsystem2/2(isInputValid) -> Sum/2
  powerLoads/1 -> thrustersToBuses/1(powerLoads)  "power bus"

== system connections/thruster_model/main_propeller_port ==
  desiredSetPoint : Inport  Unit=N
  desiredAzimuth : Inport  Port=2  Unit=deg
  Abs : Abs
  Add : Sum  Inputs=|+-
  Azimuth Dynamics1 : Subsystem
  Constant1 : Constant  Value=2
  Constant2 : Constant  Value=3
  Divide : Product
  From degrees to -180/+1 : Subsystem
  From degrees to -180/+180 : Subsystem
  Gain : Gain  Gain=286000
  Gain1 : Gain  Gain=1/100
  Gain2 : Gain  Gain=1500000
  Integrator1 : Integrator
  Power : Math  Operator=pow  SignedPower=on  SaturateOnIntegerOverflow=on
  Power1 : Math  Operator=pow  SignedPower=on  SaturateOnIntegerOverflow=on
  Saturation : Saturate  UpperLimit=100  LowerLimit=-100
  Sign : Signum
  p : Outport  Unit=W  VectorParamsAs1DForOutWhenUnconnected=off  BusOutputAsStruct=on
  thrust : Outport  Port=2  Unit=N  VectorParamsAs1DForOutWhenUnconnected=off
  azimuth : Outport  Port=3  Unit=deg  VectorParamsAs1DForOutWhenUnconnected=off  BusOutputAsStruct=on
  sensorFeedback : Outport  Port=4  Unit=deg  VectorParamsAs1DForOutWhenUnconnected=off  BusOutputAsStruct=on
  wires:
  Gain1/1 -> Add/1
  From degrees to -180/+180/1(treatedInput) -> Azimuth Dynamics1/1(Set Point)
  Add/1 -> Integrator1/1
  Saturation/1 -> Gain1/1
  Divide/1 -> thrust/1
  Power1/1 -> Gain2/1
  desiredSetPoint/1 -> Saturation/1  "thrustSetPoint"
  Power/1 -> Gain/1
  Azimuth Dynamics1/1(currentAngle 0/360) -> From degrees to -180/+1/1(desiredAzimuth)
  Gain/1 -> Divide/2  "thrust"
  From degrees to -180/+1/1(treatedInput) -> azimuth/1
  Gain2/1 -> Abs/1  "power"
  Constant2/1 -> Power1/2  "q"
  Sign/1 -> Divide/1
  Constant1/1 -> Power/2  "q"
  Abs/1 -> p/1
  desiredAzimuth/1 -> From degrees to -180/+180/1(desiredAzimuth)
  Integrator1/1 -> Power/1, Power1/1, sensorFeedback/1, Sign/1, Add/2

== system connections/thruster_model/main_propeller_starboard ==
  desiredSetPoint : Inport  Unit=N
  desiredAzimuth : Inport  Port=2  Unit=deg
  Abs : Abs
  Add : Sum  Inputs=|+-
  Azimuth Dynamics1 : Subsystem
  Constant1 : Constant  Value=2
  Constant2 : Constant  Value=3
  Divide : Product
  From degrees to -180/+1 : Subsystem
  From degrees to -180/+180 : Subsystem
  Gain : Gain  Gain=286000
  Gain1 : Gain  Gain=1/100
  Gain2 : Gain  Gain=1500000
  Integrator : Integrator
  Power : Math  Operator=pow  SignedPower=on  SaturateOnIntegerOverflow=on
  Power1 : Math  Operator=pow  SignedPower=on  SaturateOnIntegerOverflow=on
  Saturation : Saturate  UpperLimit=100  LowerLimit=-100
  Sign : Signum
  p : Outport  Unit=W  VectorParamsAs1DForOutWhenUnconnected=off  BusOutputAsStruct=on
  thrust : Outport  Port=2  Unit=N  VectorParamsAs1DForOutWhenUnconnected=off
  azimuth : Outport  Port=3  Unit=deg  VectorParamsAs1DForOutWhenUnconnected=off  BusOutputAsStruct=on
  sensorFeedback : Outport  Port=4  Unit=deg  VectorParamsAs1DForOutWhenUnconnected=off  BusOutputAsStruct=on
  wires:
  desiredAzimuth/1 -> From degrees to -180/+180/1(desiredAzimuth)
  Abs/1 -> p/1
  Constant1/1 -> Power/2  "q"
  Sign/1 -> Divide/1
  Constant2/1 -> Power1/2  "q"
  Gain2/1 -> Abs/1  "power"
  From degrees to -180/+1/1(treatedInput) -> azimuth/1
  Gain/1 -> Divide/2  "thrust"
  Azimuth Dynamics1/1(currentAngle 0/360) -> From degrees to -180/+1/1(desiredAzimuth)
  Power/1 -> Gain/1
  desiredSetPoint/1 -> Saturation/1  "thrustSetPoint"
  Power1/1 -> Gain2/1
  Divide/1 -> thrust/1
  Saturation/1 -> Gain1/1
  Add/1 -> Integrator/1
  From degrees to -180/+180/1(treatedInput) -> Azimuth Dynamics1/1(Set Point)
  Gain1/1 -> Add/1
  Integrator/1 -> Sign/1, sensorFeedback/1, Power/1, Power1/1, Add/2

== system connections/thruster_model/tunnel_thruster_1 ==
  desiredSetPoint : Inport  Unit=N
  desiredAzimuth : Inport  Port=2  Unit=deg
  Abs : Abs
  Add : Sum  Inputs=|+-
  Constant1 : Constant  Value=2
  Constant2 : Constant  Value=3
  Divide : Product
  Gain : Gain  Gain=144000
  Gain1 : Gain  Gain=1/100
  Gain2 : Gain  Gain=925000
  Integrator1 : Integrator
  Power : Math  Operator=pow  SignedPower=on  SaturateOnIntegerOverflow=on
  Power1 : Math  Operator=pow  SignedPower=on  SaturateOnIntegerOverflow=on
  Saturation : Saturate  UpperLimit=100  LowerLimit=-100
  Sign : Signum
  p : Outport  Unit=W  VectorParamsAs1DForOutWhenUnconnected=off  BusOutputAsStruct=on
  thrust : Outport  Port=2  Unit=N  VectorParamsAs1DForOutWhenUnconnected=off
  azimuth : Outport  Port=3  Unit=deg  VectorParamsAs1DForOutWhenUnconnected=off  BusOutputAsStruct=on
  sensorFeedback : Outport  Port=4  Unit=deg  VectorParamsAs1DForOutWhenUnconnected=off  BusOutputAsStruct=on
  wires:
  Abs/1 -> p/1
  Constant1/1 -> Power/2  "q"
  Sign/1 -> Divide/1
  Constant2/1 -> Power1/2  "q"
  Gain2/1 -> Abs/1  "power"
  Gain/1 -> Divide/2  "thrust"
  Power/1 -> Gain/1
  desiredSetPoint/1 -> Saturation/1  "thrustSetPoint"
  Power1/1 -> Gain2/1
  Divide/1 -> thrust/1
  Saturation/1 -> Gain1/1
  Integrator1/1 -> Add/2, Sign/1, sensorFeedback/1, Power1/1, Power/1
  Add/1 -> Integrator1/1
  Gain1/1 -> Add/1
  desiredAzimuth/1 -> azimuth/1

== system connections/thruster_model/tunnel_thruster_2 ==
  desiredSetPoint : Inport  Unit=N
  desiredAzimuth : Inport  Port=2  Unit=deg
  Abs : Abs
  Add : Sum  Inputs=|+-
  Constant1 : Constant  Value=2
  Constant2 : Constant  Value=3
  Divide : Product
  Gain : Gain  Gain=144000
  Gain1 : Gain  Gain=1/100
  Gain2 : Gain  Gain=925000
  Integrator1 : Integrator
  Power : Math  Operator=pow  SignedPower=on  SaturateOnIntegerOverflow=on
  Power1 : Math  Operator=pow  SignedPower=on  SaturateOnIntegerOverflow=on
  Saturation : Saturate  UpperLimit=100  LowerLimit=-100
  Sign : Signum
  p : Outport  Unit=W  VectorParamsAs1DForOutWhenUnconnected=off  BusOutputAsStruct=on
  thrust : Outport  Port=2  Unit=N  VectorParamsAs1DForOutWhenUnconnected=off
  azimuth : Outport  Port=3  Unit=deg  VectorParamsAs1DForOutWhenUnconnected=off  BusOutputAsStruct=on
  sensorFeedback : Outport  Port=4  Unit=deg  VectorParamsAs1DForOutWhenUnconnected=off  BusOutputAsStruct=on
  wires:
  Gain1/1 -> Add/1
  Add/1 -> Integrator1/1
  Integrator1/1 -> Add/2, Power/1, Power1/1, sensorFeedback/1, Sign/1
  Saturation/1 -> Gain1/1
  Divide/1 -> thrust/1
  Power1/1 -> Gain2/1
  desiredSetPoint/1 -> Saturation/1  "thrustSetPoint"
  Power/1 -> Gain/1
  Gain/1 -> Divide/2  "thrust"
  Gain2/1 -> Abs/1  "power"
  Constant2/1 -> Power1/2  "q"
  Sign/1 -> Divide/1
  Constant1/1 -> Power/2  "q"
  Abs/1 -> p/1
  desiredAzimuth/1 -> azimuth/1
